simulink model "P1_fuzzy_sim"  (R2015a)
settings: Solver=ode5  SolverMode=SingleTasking  StartTime=0.0  StopTime=100  FixedStep=0.01  RelTol=1e-3  AbsTol=1e-6
libraries: fuzblock x1
settings Model: SimulationMode=external  CovSFcnEnable=off  ExtModeTrigDuration=18000  ExtModeTrigLevel=0.400000  Creator=jims  LastModifiedBy=inteco
settings DataIOCC: ExternalInput=[]  InitialState=[]  LimitDataPoints=off  MaxDataPoints=5000  SignalLoggingSaveFormat=ModelDataLogs  SaveOutput=off  SaveTime=off  SignalLoggingName=sigsOut
settings OptimizationCC: BooleanDataType=off  ExpressionDepthLimit=2147483647
settings DebuggingCC: SaveWithParameterizedLinksMsg=none  UnderspecifiedInitializationDetection=Classic  MergeDetectMultiDrivingBlocksExec=none  SignalResolutionControl=TryResolveAllWithWarning  MultiTaskDSMMsg=warning  MultiTaskCondExecSysMsg=none  IntegerOverflowMsg=none  FcnCallInpInsideContextMsg=EnableAllAsWarning  StateNameClashWarn=warning  StrictBusMsg=None  IntegerSaturationMsg=none
settings HardwareCC: ProdIntDivRoundTo=Zero  ProdEndianess=LittleEndian  ProdHWDeviceType=Intel->x86/Pentium  TargetIntDivRoundTo=Zero  TargetEndianess=LittleEndian  TargetHWDeviceType=Intel->x86/Pentium
settings RTWCC: SystemTargetFile=rtwin.tlc  TemplateMakefile=pendulum1_win_vc.tmf  RTWCompilerOptimization=on
settings RTWinTargetCC: TargetPreCompLibLocation=E:\apps_W32\MATLAB\R2015a\toolbox\sldrt\lib\win32

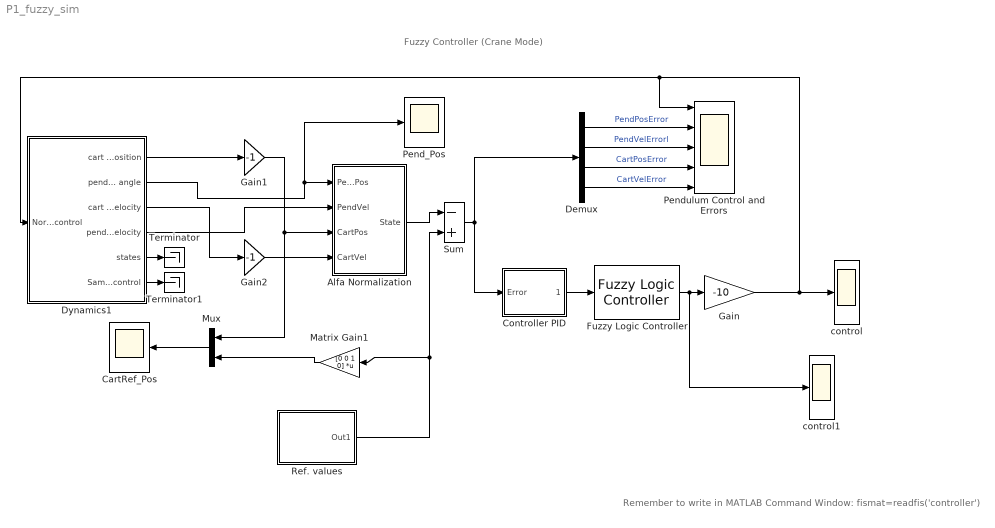
== system P1_fuzzy_sim ==
  note: Fuzzy Controller
      | (Crane Mode)
  note: Remember to write in MATLAB Command Window:
      |  fismat=readfis('controller')
  Alfa Normalization : Subsystem  mask(Choose mode:){}
  CartRef_Pos : Scope
      settings: TimeRange=60  YMin=-0.3  YMax=0.3  SaveName=Cart_refpos1  MaxDataPoints=50000
  Controller PID : Subsystem
  Demux : Demux
  Dynamics1 : Subsystem  mask(Dynamics){x_ini=[-0.25, pi, 0, 0], m=[0.5723*1.8, 0.12*2], fr=[0.00027344,  1.1975875,  0.5*2], P4=[0.01955717*0.6, 0.0038583, 9.81], Up=[ 12.86*0.5, 0.093125], DZ=[0.1, 1.5]}
      mask prompts: x_ini "Initial state vector [x1(0)  x2(0)  x3(0)  x4(0)]"; m "mass of cart (mc)  mass of pendulum (mp)"; fr "friction :  fp  FS  FC"; P4 "Distance (l), Total Inertia moment (J), gravity (g)"; Up "control : magnitude (M)    DZu"; DZ "minimal velocities : cart (DZcv)  pendulum (DZcp)"
      mask help:
      | Pendulum-Cart Dynamics
      |
      | Copyright INTECO 1997
      mask init:
      | DZcv=DZ(1);DZcp=DZ(2);DZu=Up(2);l=P4(1);J=P4(2);g=P4(3);M=Up(1);mc=m(1);mp=m(2);fp=fr(1);FS=fr(2);FC=fr(3);mi=l*(mc+mp);a=l*l+J/(mc+mp);
      mask Display: plot(0,0,100,100,[40,48,48,40,40],[60,60,49,49,60],[37,44],[9,54],[100,8,4,1,0,100,100,0,40,100,100,0,0,40],[44,44,44,44,45,46,45,44,45,45,43,43,46,46],[100,48],[55,55],[0,40],[55,55])
  Fuzzy Logic Controller : fuzblock/Fuzzy Logic  Controller  fis=fismat
  Gain : Gain  Gain=-10  SaturateOnIntegerOverflow=on  OutDataTypeStr=Inherit: Same as input  ParamDataTypeStr=Inherit: Same as input
  Gain1 : Gain  Gain=-1  SaturateOnIntegerOverflow=on  OutDataTypeStr=Inherit: Same as input  ParamDataTypeStr=Inherit: Same as input
  Gain2 : Gain  Gain=-1  SaturateOnIntegerOverflow=on  OutDataTypeStr=Inherit: Same as input  ParamDataTypeStr=Inherit: Same as input
  Matrix Gain1 : Gain  Gain=[0 0 1 0]  Multiplication=Matrix(K*u)  SaturateOnIntegerOverflow=on  OutDataTypeStr=Inherit: Same as input  ParamDataTypeStr=Inherit: Same as input
  Mux : Mux  Inputs=2
  Pend_Pos : Scope
      settings: TimeRange=60  YMin=2.975  YMax=3.3  SaveName=Cart_refpos4  MaxDataPoints=50000
  Pendulum Control and Errors : Scope  NumInputPorts=5
      settings: TimeRange=60  YMin=-0.75~-0.075~-0.5~-0.5~-0.2  YMax=0.75~0.075~0.5~0.5~0.2  SaveName=States  MaxDataPoints=50000
  Ref. values : Subsystem  mask{Sine=off, Square=on, Sawtooth=off, Amplitude=0.25, Frequency=0.02}
      mask Display: disp('Generator')
  Sum : Sum  Inputs=-+  SaturateOnIntegerOverflow=on  InputSameDT=on  OutDataTypeStr=Inherit: Same as first input
  Terminator : Terminator
  Terminator1 : Terminator
  control : Scope
      settings: TimeRange=60  YMin=-0.35  YMax=0.3  SaveName=PID_FUZZY  MaxDataPoints=50000
  control1 : Scope
      settings: TimeRange=60  YMin=-0.45  YMax=0.25  SaveName=PID_FUZZY1  MaxDataPoints=50000
  wires:
  Sum/1 -> Demux/1, Controller PID/1(Error)
  Alfa Normalization/1(State) -> Sum/1
  Demux/4 -> Pendulum Control and Errors/5  "CartVelError"
  Demux/3 -> Pendulum Control and Errors/4  "CartPosError"
  Demux/2 -> Pendulum Control and Errors/3  "PendVelErrorl"
  Demux/1 -> Pendulum Control and Errors/2  "PendPosError"
  Dynamics1/2(pendulum angle) -> Alfa Normalization/1(PendPos), Pend_Pos/1
  Dynamics1/4(pendulum velocity) -> Alfa Normalization/2(PendVel)
  Dynamics1/1(cart position) -> Gain1/1
  Dynamics1/3(cart velocity) -> Gain2/1
  Dynamics1/5(states) -> Terminator/1
  Dynamics1/6(Sampled control) -> Terminator1/1
  Fuzzy Logic Controller/1 -> Gain/1, control1/1
  Gain/1 -> Pendulum Control and Errors/1, Dynamics1/1(Normalized control), control/1
  Ref. values/1(Out1) -> Sum/2, Matrix Gain1/1
  Mux/1 -> CartRef_Pos/1
  Matrix Gain1/1 -> Mux/2
  Controller PID/1(fuzzy-input) -> Fuzzy Logic Controller/1
  Gain1/1 -> Mux/1, Alfa Normalization/3(CartPos)
  Gain2/1 -> Alfa Normalization/4(CartVel)

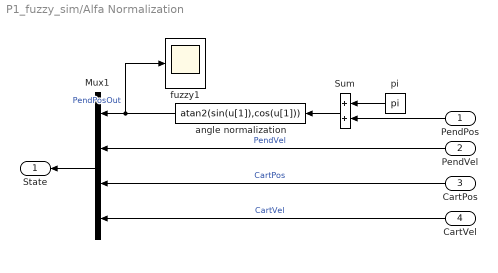
== system P1_fuzzy_sim/Alfa Normalization ==
  PendPos : Inport
  PendVel : Inport  Port=2
  CartPos : Inport  Port=3
  CartVel : Inport  Port=4
  Mux1 : Mux
  Sum : Sum  SaturateOnIntegerOverflow=on  InputSameDT=on  OutDataTypeStr=Inherit: Same as first input
  angle normalization : Fcn  Expr=atan2(sin(u[1]),cos(u[1]))
  fuzzy1 : Scope
      settings: TimeRange=60  YMin=-3.5  YMax=3.5  SaveName=Cart_refpos5  MaxDataPoints=50000
  pi : Constant  Value=pi
  State : Outport  InitialOutput=0
  wires:
  pi/1 -> Sum/1
  Sum/1 -> angle normalization/1
  Mux1/1 -> State/1
  CartPos/1 -> Mux1/3  "CartPos"
  CartVel/1 -> Mux1/4  "CartVel"
  PendVel/1 -> Mux1/2  "PendVel"
  PendPos/1 -> Sum/2
  angle normalization/1 -> Mux1/1, fuzzy1/1  "PendPosOut"

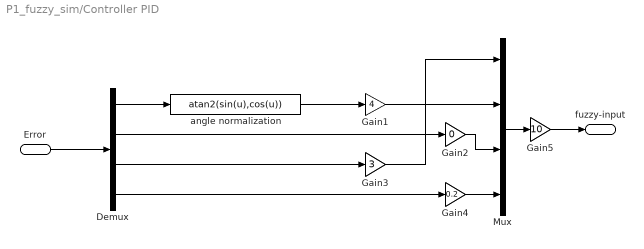
== system P1_fuzzy_sim/Controller PID ==
  Error : Inport
  Demux : Demux
  Gain1 : Gain  Gain=4  SaturateOnIntegerOverflow=on  OutDataTypeStr=Inherit: Same as input  ParamDataTypeStr=Inherit: Same as input
  Gain2 : Gain  Gain=0  SaturateOnIntegerOverflow=on  OutDataTypeStr=Inherit: Same as input  ParamDataTypeStr=Inherit: Same as input
  Gain3 : Gain  Gain=3  SaturateOnIntegerOverflow=on  OutDataTypeStr=Inherit: Same as input  ParamDataTypeStr=Inherit: Same as input
  Gain4 : Gain  Gain=0.2  SaturateOnIntegerOverflow=on  OutDataTypeStr=Inherit: Same as input  ParamDataTypeStr=Inherit: Same as input
  Gain5 : Gain  Gain=10  SaturateOnIntegerOverflow=on  OutDataTypeStr=Inherit: Same as input  ParamDataTypeStr=Inherit: Same as input
  Mux : Mux
  angle normalization : Fcn  Expr=atan2(sin(u),cos(u))
  fuzzy-input : Outport  InitialOutput=0
  wires:
  angle normalization/1 -> Gain1/1
  Gain1/1 -> Mux/2
  Demux/1 -> angle normalization/1
  Error/1 -> Demux/1
  Demux/3 -> Gain3/1
  Mux/1 -> Gain5/1
  Gain3/1 -> Mux/1
  Demux/2 -> Gain2/1
  Demux/4 -> Gain4/1
  Gain2/1 -> Mux/3
  Gain4/1 -> Mux/4
  Gain5/1 -> fuzzy-input/1

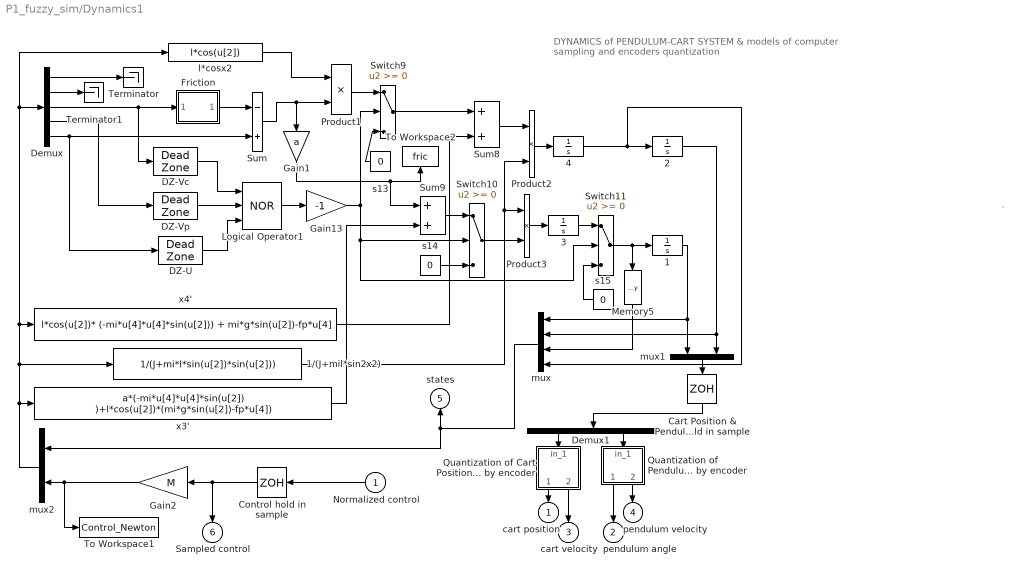
== system P1_fuzzy_sim/Dynamics1 ==
  note: DYNAMICS of
      | PENDULUM-CART SYSTEM
      | & models of
      | computer sampling and encoders quantization
  note: .
  Normalized control : Inport
  " Quantization of Pendulum Angle introduced by encoder" : Subsystem
  1 : Integrator  InitialCondition=x_ini(1)
  1/(J+mil*sin2x2) : Fcn  Expr=1/(J+mi*l*sin(u[2])*sin(u[2]))
  2 : Integrator  InitialCondition=x_ini(2)
  3 : Integrator  InitialCondition=x_ini(3)
  4 : Integrator  InitialCondition=x_ini(4)
  Cart Position & Pendulum Angle hold in sample : ZeroOrderHold  SampleTime=0.01
  Control hold in sample : ZeroOrderHold  SampleTime=0.01
  DZ-U : DeadZone  LowerValue=-DZu  UpperValue=DZu  SaturateOnIntegerOverflow=on
  DZ-Vc : DeadZone  LowerValue=-DZcv  UpperValue=DZcv  SaturateOnIntegerOverflow=on
  DZ-Vp : DeadZone  LowerValue=-DZcp  UpperValue=DZcp  SaturateOnIntegerOverflow=on
  Demux : Demux  Outputs=5
  Demux1 : Demux  Outputs=2
  Friction : Subsystem  mask(Coulombic and Viscous Friction){FS=FS, FC=FC}
      mask prompts: FS "Static friction"; FC "Coulomb friction"
      mask help:
      | A discontinuity offset at zero models coulomb friction.  Linear gain models viscous friction.
      | y = sign(x) * (Umax * abs(x) + friction)
      mask Help:
      | This block has a discontinuity
      | at zero and a linear gain afterward.
      | y= sign(x)*(Umax*abs(x)+friction)
  Gain1 : Gain  Gain=a  SaturateOnIntegerOverflow=on  OutDataTypeStr=Inherit: Same as input  ParamDataTypeStr=Inherit: Same as input
  Gain13 : Gain  Gain=-1  SaturateOnIntegerOverflow=on  OutDataTypeStr=Inherit: Same as input  ParamDataTypeStr=Inherit: Same as input
  Gain2 : Gain  Gain=M  SaturateOnIntegerOverflow=on  OutDataTypeStr=Inherit: Same as input  ParamDataTypeStr=Inherit: Same as input
  Logical Operator1 : Logic  Operator=NOR  Inputs=3
  Memory5 : Memory
  Product1 : Product  SaturateOnIntegerOverflow=on  InputSameDT=on  OutDataTypeStr=Inherit: Same as first input
  Product2 : Product  SaturateOnIntegerOverflow=on  InputSameDT=on  OutDataTypeStr=Inherit: Same as first input
  Product3 : Product  SaturateOnIntegerOverflow=on  InputSameDT=on  OutDataTypeStr=Inherit: Same as first input
  "Quantization of Cart Position introduced by encoder " : Subsystem
  Sum : Sum  Inputs=-+  SaturateOnIntegerOverflow=on  InputSameDT=on  OutDataTypeStr=Inherit: Same as first input
  Sum8 : Sum  SaturateOnIntegerOverflow=on  InputSameDT=on  OutDataTypeStr=Inherit: Same as first input
  Sum9 : Sum  SaturateOnIntegerOverflow=on  InputSameDT=on  OutDataTypeStr=Inherit: Same as first input
  Switch10 : Switch  SaturateOnIntegerOverflow=on  InputSameDT=on
  Switch11 : Switch  SaturateOnIntegerOverflow=on  InputSameDT=on
  Switch9 : Switch  SaturateOnIntegerOverflow=on  InputSameDT=on
  Terminator : Terminator
  Terminator1 : Terminator
  To Workspace1 : ToWorkspace  VariableName=Control_Newton
      settings: MaxDataPoints=100000
  To Workspace2 : ToWorkspace  VariableName=fric
      settings: MaxDataPoints=100000
  l*cosx2 : Fcn  Expr=l*cos(u[2])
  mux : Mux
  mux1 : Mux  Inputs=2
  mux2 : Mux  Inputs=[4 1]
  s13 : Constant  Value=0
  s14 : Constant  Value=0
  s15 : Constant  Value=0
  x3' : Fcn  Expr=a*(-mi*u[4]*u[4]*sin(u[2]) )+l*cos(u[2])*(mi*g*sin(u[2])-fp*u[4])
  x4' : Fcn  Expr=l*cos(u[2])* (-mi*u[4]*u[4]*sin(u[2])) + mi*g*sin(u[2])-fp*u[4]
  cart position : Outport  InitialOutput=0
  pendulum angle : Outport  Port=2  InitialOutput=0
  cart velocity : Outport  Port=3  InitialOutput=0
  pendulum velocity : Outport  Port=4  InitialOutput=0
  states : Outport  Port=5  InitialOutput=0
  Sampled control : Outport  Port=6  InitialOutput=0
  wires:
  Demux1/1 -> "Quantization of Cart Position introduced by encoder "/1(in_1)
  mux/1 -> mux2/1, states/1
  "Quantization of Cart Position introduced by encoder "/1(out_1) -> cart position/1
  "Quantization of Cart Position introduced by encoder "/2(out_2) -> cart velocity/1
  " Quantization of Pendulum Angle introduced by encoder"/1(out_1) -> pendulum angle/1
  " Quantization of Pendulum Angle introduced by encoder"/2(out_2) -> pendulum velocity/1
  Demux1/2 -> " Quantization of Pendulum Angle introduced by encoder"/1(in_1)
  Control hold in sample/1 -> Sampled control/1, Gain2/1
  Normalized control/1 -> Control hold in sample/1
  Cart Position & Pendulum Angle hold in sample/1 -> Demux1/1
  mux1/1 -> Cart Position & Pendulum Angle hold in sample/1
  1/1 -> mux1/1, mux/1
  2/1 -> mux1/2, mux/2
  4/1 -> mux/4, 2/1
  Switch11/1 -> Memory5/1, 1/1
  Memory5/1 -> mux/3
  Demux/2 -> Terminator1/1
  Demux/5 -> DZ-U/1, Sum/2
  Demux/1 -> Terminator/1
  Demux/4 -> DZ-Vp/1
  Demux/3 -> DZ-Vc/1, Friction/1(In1)
  DZ-U/1 -> Logical Operator1/3
  Logical Operator1/1 -> Gain13/1
  DZ-Vp/1 -> Logical Operator1/2
  DZ-Vc/1 -> Logical Operator1/1
  l*cosx2/1 -> Product1/1
  s13/1 -> Switch9/3
  Switch9/1 -> Sum8/1
  s14/1 -> Switch10/3
  Product1/1 -> Switch9/1
  x4'/1 -> Sum8/2
  Sum8/1 -> Product2/1
  Product2/1 -> 4/1
  Product3/1 -> 3/1
  Sum9/1 -> Switch10/1
  3/1 -> Switch11/1
  s15/1 -> Switch11/3
  Gain13/1 -> Switch9/2, Switch11/2, Switch10/2
  Switch10/1 -> Product3/2
  Sum/1 -> Product1/2, Gain1/1
  mux2/1 -> x3'/1, Demux/1, l*cosx2/1, x4'/1, 1/(J+mil*sin2x2)/1
  x3'/1 -> Sum9/2
  1/(J+mil*sin2x2)/1 -> Product2/2, Product3/1
  Gain1/1 -> Sum9/1, To Workspace2/1
  Gain2/1 -> To Workspace1/1, mux2/2
  Friction/1(Out1) -> Sum/1

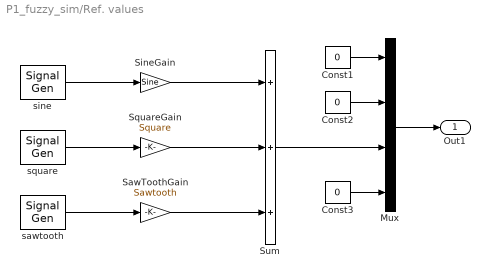
== system P1_fuzzy_sim/Ref. values ==
  Const1 : Constant  Value=0
  Const2 : Constant  Value=0
  Const3 : Constant  Value=0
  Mux : Mux
  SawToothGain : Gain  Gain=Sawtooth  SaturateOnIntegerOverflow=on  OutDataTypeStr=Inherit: Same as input  ParamDataTypeStr=Inherit: Same as input
  SineGain : Gain  Gain=Sine  SaturateOnIntegerOverflow=on  OutDataTypeStr=Inherit: Same as input  ParamDataTypeStr=Inherit: Same as input
  SquareGain : Gain  Gain=Square  SaturateOnIntegerOverflow=on  OutDataTypeStr=Inherit: Same as input  ParamDataTypeStr=Inherit: Same as input
  Sum : Sum  Inputs=+++  SaturateOnIntegerOverflow=on  InputSameDT=on  OutDataTypeStr=Inherit: Same as first input
  sawtooth : SignalGenerator  WaveForm=sawtooth  Amplitude=Amplitude  Frequency=Frequency
  sine : SignalGenerator  Amplitude=Amplitude  Frequency=Frequency
  square : SignalGenerator  WaveForm=square  Amplitude=Amplitude  Frequency=Frequency
  Out1 : Outport  InitialOutput=0
  wires:
  Mux/1 -> Out1/1
  Const3/1 -> Mux/4
  Const2/1 -> Mux/2
  Const1/1 -> Mux/1
  Sum/1 -> Mux/3
  sine/1 -> SineGain/1
  square/1 -> SquareGain/1
  sawtooth/1 -> SawToothGain/1
  SineGain/1 -> Sum/1
  SquareGain/1 -> Sum/2
  SawToothGain/1 -> Sum/3

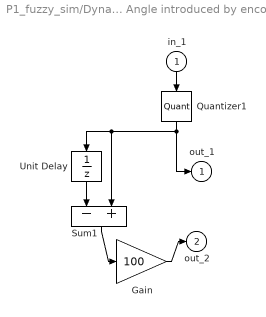
== system P1_fuzzy_sim/Dynamics1/ Quantization of Pendulum Angle introduced by encoder ==
  in_1 : Inport
  Gain : Gain  Gain=100  SaturateOnIntegerOverflow=on  OutDataTypeStr=Inherit: Same as input  ParamDataTypeStr=Inherit: Same as input
  Quantizer1 : Quantizer  QuantizationInterval=5.7053e-005
  Sum1 : Sum  Inputs=-+  SaturateOnIntegerOverflow=on  InputSameDT=on  OutDataTypeStr=Inherit: Same as first input
  Unit Delay : UnitDelay  InitialCondition=x_ini(2)  SampleTime=0.01
  out_1 : Outport  InitialOutput=0
  out_2 : Outport  Port=2  InitialOutput=0
  wires:
  in_1/1 -> Quantizer1/1
  Quantizer1/1 -> Sum1/2, Unit Delay/1, out_1/1
  Sum1/1 -> Gain/1
  Gain/1 -> out_2/1
  Unit Delay/1 -> Sum1/1

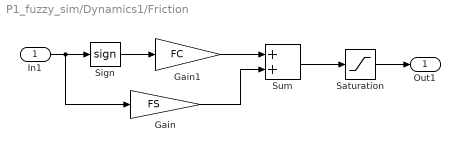
== system P1_fuzzy_sim/Dynamics1/Friction ==
  In1 : Inport
  Gain : Gain  Gain=FS  SaturateOnIntegerOverflow=on  OutDataTypeStr=Inherit: Same as input  ParamDataTypeStr=Inherit: Same as input
  Gain1 : Gain  Gain=FC  SaturateOnIntegerOverflow=on  OutDataTypeStr=Inherit: Same as input  ParamDataTypeStr=Inherit: Same as input
  Saturation : Saturate  UpperLimit=1  LowerLimit=-1
  Sign : Signum
  Sum : Sum  SaturateOnIntegerOverflow=on  InputSameDT=on  OutDataTypeStr=Inherit: Same as first input
  Out1 : Outport  InitialOutput=0
  wires:
  Saturation/1 -> Out1/1
  Sum/1 -> Saturation/1
  Sign/1 -> Gain1/1
  In1/1 -> Gain/1, Sign/1
  Gain1/1 -> Sum/1
  Gain/1 -> Sum/2

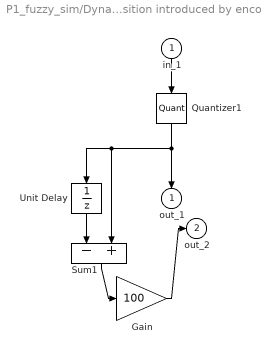
== system P1_fuzzy_sim/Dynamics1/Quantization of Cart Position introduced by encoder  ==
  in_1 : Inport
  Gain : Gain  Gain=100  SaturateOnIntegerOverflow=on  OutDataTypeStr=Inherit: Same as input  ParamDataTypeStr=Inherit: Same as input
  Quantizer1 : Quantizer  QuantizationInterval=5.7053e-005
  Sum1 : Sum  Inputs=-+  SaturateOnIntegerOverflow=on  InputSameDT=on  OutDataTypeStr=Inherit: Same as first input
  Unit Delay : UnitDelay  InitialCondition=x_ini(1)  SampleTime=0.01
  out_1 : Outport  InitialOutput=0
  out_2 : Outport  Port=2  InitialOutput=0
  wires:
  Quantizer1/1 -> Sum1/2, Unit Delay/1, out_1/1
  Unit Delay/1 -> Sum1/1
  Gain/1 -> out_2/1
  in_1/1 -> Quantizer1/1
  Sum1/1 -> Gain/1
